simulink model "Function_Call"  (R2018b)
settings: Solver=FixedStepDiscrete  StartTime=0.0  StopTime=10.0  RelTol=1e-3
settings Model: Creator=Peter Ghali  LastModifiedBy=Peter Ghali
settings OptimizationCC: DefaultParameterBehavior=Inlined  EnhancedBackFolding=on  PassReuseOutputArgsAs=Individual arguments  OptimizeBlockOrder=speed  DifferentSizesBufferReuse=on  OptimizationCustomize=off
settings DebuggingCC: ParameterTunabilityLossMsg=error
settings SFSimCC: MATLABDynamicMemAlloc=off
settings RTWCC: SystemTargetFile=ert.tlc  GenCodeOnly=on  TemplateMakefile=ert_default_tmf  GenerateReport=on  IncludeHyperlinkInReport=on  LaunchReport=on  GenerateTraceInfo=on  GenerateTraceReport=on  GenerateTraceReportSl=on  GenerateTraceReportSf=on  GenerateTraceReportEml=on
settings CodeAppCC: ForceParamTrailComments=on  IgnoreCustomStorageClasses=off  OperatorAnnotations=on  SimulinkDataObjDesc=on  SFDataObjDesc=on  InsertBlockDesc=on
settings ERTTargetCC: TargetLangStandard=C99 (ISO)  GenerateSampleERTMain=on  InlinedParameterPlacement=NonHierarchical  ERTCustomFileTemplate=example_file_process.tlc

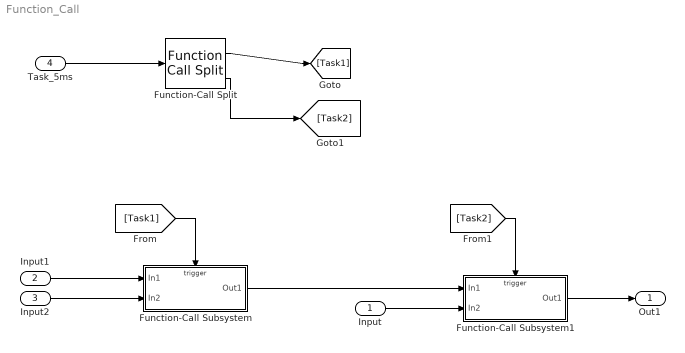
== system Function_Call ==
  Input : Inport
  Input1 : Inport  Port=2
  Input2 : Inport  Port=3
  Task_5ms : Inport  Port=4  OutputFunctionCall=on
  Function-Call Split : FunctionCallSplit  NumOutputPorts=2  OutputPortLayout=default
  Function-Call Subsystem : Subsystem  TreatAsAtomicUnit=on  RTWFcnName=Add_Function
      settings: RTWFcnNameOpts=User specified
  Function-Call Subsystem1 : Subsystem  TreatAsAtomicUnit=on  RTWFcnName=Sub_Function
      settings: RTWFcnNameOpts=User specified
  Out1 : Outport
  wires:
  Function-Call Subsystem/1(Out1) -> Function-Call Subsystem1/1(In1)
  Input/1 -> Function-Call Subsystem1/2(In2)
  Input2/1 -> Function-Call Subsystem/2(In2)
  Input1/1 -> Function-Call Subsystem/1(In1)
  Function-Call Subsystem1/1(Out1) -> Out1/1
  Task_5ms/1 -> Function-Call Split/1
  Function-Call Split/1 -> [Task1]
  [Task1] -> Function-Call Subsystem/Trigger
  Function-Call Split/2 -> [Task2]
  [Task2] -> Function-Call Subsystem1/Trigger

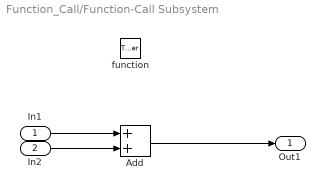
== system Function_Call/Function-Call Subsystem ==
  In1 : Inport
  In2 : Inport  Port=2
  function : TriggerPort  TriggerType=function-call  VariantControl=Variant
  Add : Sum
  Out1 : Outport
  wires:
  In1/1 -> Add/1
  Add/1 -> Out1/1
  In2/1 -> Add/2

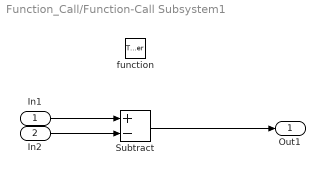
== system Function_Call/Function-Call Subsystem1 ==
  In1 : Inport
  In2 : Inport  Port=2
  function : TriggerPort  TriggerType=function-call  VariantControl=Variant
  Subtract : Sum  Inputs=+-
  Out1 : Outport
  wires:
  In1/1 -> Subtract/1
  Subtract/1 -> Out1/1
  In2/1 -> Subtract/2
